simulink model "nav3v2"  (R2020a)
settings: Solver=FixedStepAuto  StartTime=0.0  StopTime=inf  RelTol=1e-3
model workspace (MAT data in the model file):
  SL_ROS_VariableLengthArrays_MaxSizes : object (value not decoded)
values from neighbouring files (symbols this model uses):
  map = binaryOccupancyMap(logicalMap, 1/0.05)    [exampleHelperVisualizeExecuteRobots.m]
undefined symbols (not defined in the file or in its folder): Angular, Data, Data_SL_Info, gray, Linear
libraries: robotlib x47, simulink x1
(part 2 of 2)

== stateflow chart nav3v2/Control_Subsystem/State_Machine ==
  state atGoal = checkAtGoal(pose,goalWaypoint,goalTolerance) [function]
  state angVel = PID(pose,desiredHeading,P,I,D) [function]
  state INITIALISATION
    entry:
    currentState = INITIALISATION_STATE;
  state WAITING
    entry:
    currentState = WAITING_STATE;
    during:
    linearVel = 0;
    angularVel = 0;
  state REVERSE
    state RotateToWaypoint
      entry:
      % Set currentState
      currentState = REVERSE_STATE + 1;
      waypointLinePID = all_waypoints(count:count+1,:);
      % Set linear velocity to zero and calculate goal heading
      linearVel = 0;
      currentGoalHeading = CalculateHeading(currentPose, all_waypoints(count+1,:));
      goalHeading = [currentGoalHeading; 0; 0];
      during:
      % Try and reach that goal heading
      angularVel = PID(currentPose, goalHeading(1,1), P, I, D);
      % Zero out angular velocity
      exit:
      angularVel = 0;
    state MoveToWaypoint
      entry:
      currentState = REVERSE_STATE + 3;
      linearVel = MAX_LINEAR_VEL/2;
      during:
      goalHeading = purePursuit(LOOKAHEAD_DISTANCE, MAX_LINEAR_VEL, ...
      MAX_ANGULAR_VEL, waypointLinePID, currentPose);
      angularVel = PID(currentPose, goalHeading(1,1), P, I, D);
    state PreciseMoveToWaypoint
      currentState = REVERSE_STATE + 4;
      linearVel = MAX_LINEAR_VEL/2;
      during:
      currentGoalHeading = CalculateHeading(currentPose, all_waypoints(count+1,:));
      goalHeading = [currentGoalHeading; 0; 0];
      angularVel = PID(currentPose, goalHeading(1,1), P, I, D);
    state ReachedWaypoint
      entry:
      currentState = REVERSE_STATE + 5;
    (default) -> REVERSE.RotateToWaypoint : {currentState = REVERSE_STATE;
        | all_waypoints = [currentPose(1:2,:)'; waypointList];
        | [last, ~] = size(all_waypoints);
        | finishedMissionCount = 0;
        | finishedMission = 0;
        | count = 1;}
    (junction 329) -> REVERSE.RotateToWaypoint [order 2] : [mod(finishedMissionCount, 2) == 0]
        | {all_waypoints = [currentPose(1:2,:)'; waypointList];}
    REVERSE.ReachedWaypoint -> REVERSE.RotateToWaypoint [order 2] : [count+1 < last]
        | {count =  count + 1;}
    REVERSE.RotateToWaypoint -> MoveToWaypoint : [currentGoalHeading - 0.01< currentPose(3) && currentPose(3) < currentGoalHeading + 0.01]
    (junction 329) -> REVERSE.RotateToWaypoint [order 1] : [mod(finishedMissionCount, 2) == 1]
        | {all_waypoints = [flip(waypointList); currentPose(1:2,:)'];}
    REVERSE.ReachedWaypoint -> (junction 329) [order 1] : [count + 1 == last]
        | {finishedMissionCount = finishedMissionCount + 1;
        | count = 1;}
    MoveToWaypoint -> REVERSE.PreciseMoveToWaypoint : [~checkAtGoal(currentPose, all_waypoints(count+1,:)', LOOKAHEAD_DISTANCE)]
    REVERSE.PreciseMoveToWaypoint -> REVERSE.ReachedWaypoint : [~checkAtGoal(currentPose, all_waypoints(count+1,:)', WAYPOINT_PRECISION)]
  state AUTONOMOUS_CONTROL
    state RotateToWaypoint
      entry:
      % Set currentState
      currentState = AUTONOMOUS_CONTROL_STATE + 1;
      % Set linear velocity to zero and calculate goal heading
      linearVel = 0;
      currentGoalHeading = CalculateHeading(currentPose, all_waypoints(count+1,:));
      goalHeading = [currentGoalHeading; 0; 0];
      during:
      % Try and reach that goal heading
      angularVel = PID(currentPose, goalHeading(1,1), P, I, D);
      % Zero out angular velocity
      exit:
      angularVel = 0;
    state PurePursuitMoveToWaypoint
      entry:
      currentState = AUTONOMOUS_CONTROL_STATE + 2;
      during:
      % Calculate the goal heaing using pure pursuit
      goalHeading = purePursuit(LOOKAHEAD_DISTANCE, MAX_LINEAR_VEL, ...
      MAX_ANGULAR_VEL, waypointLine, currentPose);
      % Set Linear and Angular Speeds
      linearVel = MAX_LINEAR_VEL;
      angularVel = PID(currentPose, goalHeading(1,1), P, I, D);
      % Log Current waypoint
      currentWaypoint = all_waypoints(count+1,:)';
    state PreciseRotateToWaypoint
      entry:
      currentState = AUTONOMOUS_CONTROL_STATE + 1;
      % Set linear velocity to zero and calculate goal heading
      linearVel = 0;
      currentGoalHeading = CalculateHeading(currentPose, all_waypoints(count+1,:));
      currentWaypoint = all_waypoints(count+1,:)';
      during:
      % Try and reach that goal heading
      angularVel = PID(currentPose, currentGoalHeading(1,1), P, I, D);
      % Zero out angular velocity
      exit:
      angularVel = 0;
    state PreciseMoveToWaypoint
      entry:
      currentState = AUTONOMOUS_CONTROL_STATE + 3;
      linearVel = MAX_LINEAR_VEL/2;
      during:
      currentGoalHeading = CalculateHeading(currentPose, all_waypoints(count+1,:));
      angularVel = PID(currentPose, currentGoalHeading(1,1), P, I, D);
    state ReachedWaypoint
      entry:
      currentState = AUTONOMOUS_CONTROL_STATE + 4;
    (default) -> AUTONOMOUS_CONTROL.RotateToWaypoint : {currentState = AUTONOMOUS_CONTROL_STATE;
        | all_waypoints = [currentPose(1:2,:)'; waypointList];
        | [last, ~] = size(all_waypoints);
        | finishedMissionCount = 0;
        | finishedMission = 0;
        | count = 1;}
    (junction 225) -> AUTONOMOUS_CONTROL.RotateToWaypoint [order 2] : [mod(finishedMissionCount, 2) == 0]
        | {all_waypoints = [currentPose(1:2,:)'; waypointList];}
    AUTONOMOUS_CONTROL.RotateToWaypoint -> (junction 203) : [currentGoalHeading - 0.01< currentPose(3) && currentPose(3) < currentGoalHeading + 0.01]
    (junction 225) -> AUTONOMOUS_CONTROL.RotateToWaypoint [order 1] : [mod(finishedMissionCount, 2) == 1]
        | {all_waypoints = [flip(waypointList); currentPose(1:2,:)'];}
    (junction 203) -> PurePursuitMoveToWaypoint [order 2] : [count + 2 <= last]
        | {waypointLine = all_waypoints(count:count+2, 1:2);}
    (junction 203) -> PreciseRotateToWaypoint [order 1] : [count + 2 > last]
        | {waypointLine = [currentPose(1:2,:)'; all_waypoints(count:count+1,1:2)];}
    AUTONOMOUS_CONTROL.ReachedWaypoint -> (junction 203) [order 1] : [count+1 < last]
        | {count =  count + 1;}
    AUTONOMOUS_CONTROL.ReachedWaypoint -> (junction 225) [order 2] : [count + 1 == last]
        | {finishedMissionCount = finishedMissionCount + 1;
        | count = 1;}
    PurePursuitMoveToWaypoint -> AUTONOMOUS_CONTROL.ReachedWaypoint : [~checkAtGoal(currentPose, all_waypoints(count+1,:)', LOOKAHEAD_DISTANCE)]
    PreciseRotateToWaypoint -> AUTONOMOUS_CONTROL.PreciseMoveToWaypoint : [currentGoalHeading - 0.01< currentPose(3) && currentPose(3) < currentGoalHeading + 0.01]
    AUTONOMOUS_CONTROL.PreciseMoveToWaypoint -> AUTONOMOUS_CONTROL.ReachedWaypoint : [~checkAtGoal(currentPose, all_waypoints(count+1,:)', WAYPOINT_PRECISION)]
  state MANUAL_CONTROL
    entry:
    currentState = MANUAL_CONTROL_STATE;
    during:
    angularVel = joystickAngularVel;
    linearVel = joystickLinearVel;
  state EMERGENCY
    entry:
    currentState = EMERGENCY_STATE;
    during:
    linearVel = 0;
    angularVel = 0;
  (default) -> INITIALISATION
  INITIALISATION -> WAITING
  WAITING -> REVERSE [order 3] : [reverseButton == 1]
  REVERSE -> EMERGENCY [order 1] : [emergencyButton == 1]
  WAITING -> AUTONOMOUS_CONTROL [order 4] : [missionStartButton == 1]
  REVERSE -> WAITING [order 2] : [waitingButton == 1]
  AUTONOMOUS_CONTROL -> WAITING [order 2] : [waitingButton == 1]
  AUTONOMOUS_CONTROL -> WAITING [order 3] : [finishedMission == 1]
  WAITING -> MANUAL_CONTROL [order 1] : [manualControlButton == 1]
  AUTONOMOUS_CONTROL -> EMERGENCY [order 1] : [emergencyButton == 1]
  MANUAL_CONTROL -> WAITING [order 2] : [waitingButton == 1]
  WAITING -> EMERGENCY [order 2] : [emergencyButton == 1]
  EMERGENCY -> WAITING : [restoreEStopButton == 1]
  MANUAL_CONTROL -> EMERGENCY [order 1] : [emergencyButton == 1]
  data: lookAhead function_input; maxLinVel function_input; maxAngVel function_input; waypoints function_input; pose function_input; targetHeading function_output; pose function_input double size=3; goalWaypoint function_input double size=2; atGoal function_output boolean size=1; goalTolerance function_input double size=1; angVel function_output; pose function_input double size=3; desiredHeading function_input double size=1; P function_input double size=1; I function_input double size=1; D function_input double size=1; startPose function_input; endPose function_input; heading function_output; startPose function_input; endPose function_input; heading function_output; currentPose input size=3; voltage input; missionStartButton input size=1; emergencyButton input; reverseButton input; restoreEStopButton input; currentWaypoint output size=[2 1]; currentState output size=1; linearVel output size=1; angularVel output size=1; WAITING_STATE data_store_memory; REVERSE_STATE data_store_memory; MANUAL_CONTROL_STATE data_store_memory; INITIALISATION_STATE data_store_memory; EMERGENCY_STATE data_store_memory; AUTONOMOUS_CONTROL_STATE data_store_memory; manualControlButton input; waitingButton input; joystickAngularVel input; joystickLinearVel input; LOOKAHEAD_DISTANCE data_store_memory; MAX_LINEAR_VEL data_store_memory; MAX_ANGULAR_VEL data_store_memory; D data_store_memory; P data_store_memory; I data_store_memory; goalHeading data_store_memory; waypointList input; last local; finishedMission local; finished local; count local; currentGoalHeading local; waypointLine local size=[3 2]; rotateFlag local; WAYPOINT_PRECISION data_store_memory; waypointDistance local; reversePose local size=[3 1] =[0; 0; -pi/2]; all_waypoints local; finishedMissionCount local; waypointLinePID local
  function targetHeading = purePursuit(lookAhead, maxLinVel, maxAngVel, waypoints, pose):
    | function targetHeading = purePursuit(lookAhead, maxLinVel, maxAngVel, waypoints, pose)
    | 
    |     controller = controllerPurePursuit('Waypoints', waypoints, 'LookaheadDistance', lookAhead, 'MaxAngularVelocity', maxAngVel, 'DesiredLinearVelocity', maxLinVel);
    |     
    |    [~, ~, xy] = controller(pose); 
    |    
    |    heading = atan2((xy(1,2) - pose(2,1)), (xy(1,1) - pose(1,1))); 
    |    
    |    targetHeading = [heading; xy'];
  function heading = CalculateHeading(startPose, endPose):
    | function heading = CalculateHeading(startPose, endPose)
    |    
    |    heading = atan2((endPose(1,2) - startPose(2,1)),(endPose(1,1) - startPose(1,1))); 
    |   
    | end
  function heading = CalculateReverseHeading(startPose, endPose):
    | function heading = CalculateReverseHeading(startPose, endPose)
    |    
    |    heading = atan2((startPose(2,1) - endPose(1,2)),(startPose(1,1) - endPose(1,1))); 
    |   
    | end

== matlab function nav3v2/Perception_Subsystem/SLAM_Subsystem/Live_Pose_Parser/World to Robot Transform ==
  data: pose input; robotPose output; W2ORTransform input; L2RTransform input
function robotPose = fcn(pose, W2ORTransform, L2RTransform)
    
    % W2LOTransform 
    W2LOTransform = W2ORTransform/(L2RTransform); 
    
    %LO2 Transform 
    LO2LTransform = [cos(pose(3,1)), -sin(pose(3,1)), pose(1,1);
                    sin(pose(3,1)), cos(pose(3,1)), pose(2,1);
                    0,              0,              1];

    % Calculate W2R = W2LO * LO2L * L2R
    W2RTransform = W2LOTransform*LO2LTransform*L2RTransform; 
    
    % Create 3D Rotation matrix
    rotm = [W2RTransform(1,1), W2RTransform(1,2), 0;
            W2RTransform(2,1), W2RTransform(2,2), 0; 
            0                , 0                , 1;]; 
    
    % Extract axis angle
    quat = rotm2quat(rotm);
    heading = quat2eul(quat); 
    
robotPose = [W2RTransform(1,3); W2RTransform(2,3); heading(1,1)];

== matlab function nav3v2/Perception_Subsystem/SLAM_Subsystem/Map_2_Image ==
  data: map input; image output size=[1000,1000]
function image = fcn(map)

image = imcomplement(flipud(map));

== matlab function nav3v2/Perception_Subsystem/IMU_Subsystem/Live_Pose_Parser/Quaternion_2_Euler ==
  data: x input; theta output; y input; z input; w input
function theta = fcn(x, y, z, w)

    euler = quat2eul([x, y, z, w]); 
    
    if sum(isnan(euler)) == 3
        
        euler = ([pi, 0, 0]);
        
    end 
    
theta = euler(1,3);

== matlab function nav3v2/Perception_Subsystem/SLAM_Subsystem/Live_Pose_Parser/Quaternion_2_Euler ==
  data: x input; theta output; y input; z input; w input
function theta = fcn(x, y, z, w)

    euler = quat2eul([x, y, z, w]); 
    
    if sum(isnan(euler)) == 3
        
        euler = ([pi, 0, 0]);
        
    end 
    
theta = euler(1,3);

== matlab function nav3v2/Parameter_Server_Subsystem/Robot_Parameters/MATLAB Function ==
  data: Lidar2RobotX input; Lidar2Robot output; Lidar2RobotY input; Lidar2RobotTheta input
function Lidar2Robot = fcn(Lidar2RobotX, Lidar2RobotY, Lidar2RobotTheta)
    
    Lidar2Robot = [cos(Lidar2RobotTheta), -sin(Lidar2RobotTheta), Lidar2RobotX;
                   sin(Lidar2RobotTheta), cos(Lidar2RobotTheta), Lidar2RobotY; 
                   0, 0, 1;];

== matlab function nav3v2/Parameter_Server_Subsystem/Experiment_Parameters/MATLAB Function ==
  data: initialPose input; World2RobotOdom output
function World2RobotOdom = fcn(initialPose)

    initialPoseX = initialPose(1,1); 
    initialPoseY = initialPose(2,1); 
    initialPoseTheta = initialPose(3,1); 

    World2RobotOdom = [cos(initialPoseTheta), -sin(initialPoseTheta), initialPoseX; 
                    sin(initialPoseTheta), cos(initialPoseTheta), initialPoseY; 
                    0            , 0            , 1];

== matlab function nav3v2/Perception_Subsystem/IMU_Subsystem/Live_Pose_Parser/TrueNorthToIMU1 ==
  data: orientation input; heading output; trueNorthAngle input
function heading = fcn(orientation, trueNorthAngle)


    % After testing 
    heading = orientation + trueNorthAngle; 
    
    % Ensure it is wrapped. 
    if heading >= pi 
        heading = heading - 2*pi; 
    elseif heading < -pi
        heading = heading + 2*pi; 
    end

== matlab function nav3v2/Perception_Subsystem/Camera_Subsystem/MATLAB Function ==
  data: image input; y output
function y = fcn(image)
    
    tagFamily = ['tag36h11']; 
    
    [id,loc,detectedFamily] = readAprilTag(image,tagFamily);
    
y = I;

== matlab function nav3v2/Perception_Subsystem/IMU_Subsystem/Live_Pose_Parser/TrueNorthToIMU ==
  data: orientation input; heading output
function heading = fcn(orientation)


    % After testing 
    heading = orientation + 1.99; 
    
    % Ensure it is wrapped. 
    if heading >= pi 
        heading = heading - 2*pi; 
    elseif heading < -pi
        heading = heading + 2*pi; 
    end

== matlab function nav3v2/Perception_Subsystem/IMU_Subsystem/Live_Pose_Parser/IMUToGround ==
  data: orientation input; heading output; trueNorthAngle input; initialPose input
function heading = fcn(orientation, trueNorthAngle, initialPose)

    % After testing 
    heading = orientation - trueNorthAngle + initialPose(3,1) ; 
    
    % Ensure it is wrapped. 
    if heading >= pi 
        heading = heading - 2*pi; 
    elseif heading < -pi
        heading = heading + 2*pi; 
    end

== matlab function nav3v2/Control_Subsystem/State_Machine/PID/Calculate_Error ==
  data: goalHeading input; currentHeading input; error output
function error = fcn(goalHeading, currentHeading)
    
    % Calculate basic error
    error = goalHeading - currentHeading;
    
    % Calculate angle wrap
    if error < -pi
        error = error + 2*pi;
    elseif error > pi
        error = (error - 2*pi);
    end

== matlab function nav3v2/Control_Subsystem/State_Machine/PID/Normalise_Heading ==
  data: headingAngle input; bearingAngle output
function bearingAngle = fcn(headingAngle)
 
    if headingAngle < 0
        headingAngle = pi + (pi - abs(headingAngle)); 
    end

bearingAngle = headingAngle;

== matlab function nav3v2/Control_Subsystem/State_Machine/PID/Normalise_Goal_Heading ==
  data: headingAngle input; bearingAngle output
function bearingAngle = fcn(headingAngle)
 
    if headingAngle < 0
        headingAngle = pi + (pi - abs(headingAngle)); 
    end

bearingAngle = headingAngle;
